simulink model "RBG_Einmassenmodell_Verifikation_Validierung"  (R2021a)
settings: Solver=ode45  StartTime=0.0  StopTime=20  MaxStep=0.02  RelTol=1e-3  EnableMultiTasking=on
settings Model: Creator=beck  LastModifiedBy=Benjamin
settings SolverCC: AlgebraicLoopSolver=TrustRegion
settings DataIOCC: LimitDataPoints=on  SaveFormat=Array  SignalLoggingSaveFormat=ModelDataLogs  ReturnWorkspaceOutputs=off
settings OptimizationCC: ExpressionDepthLimit=2147483647  InitFltsAndDblsToZero=on  LifeSpan=inf
settings DebuggingCC: SaveWithParameterizedLinksMsg=none  UnderspecifiedInitializationDetection=Classic  MergeDetectMultiDrivingBlocksExec=none  SignalResolutionControl=TryResolveAllWithWarning  SolverPrmCheckMsg=warning  FcnCallInpInsideContextMsg=warning  StateNameClashWarn=warning  SFUnexpectedBacktrackingDiag=warning  SFNoUnconditionalDefaultTransitionDiag=warning  SFExecutionAtInitializationDiag=none  SFMachineParentedDataDiag=warning  ArithmeticOperatorsInVariantConditions=warning
settings HardwareCC: ProdBitPerPointer=32  ProdBitPerSizeT=32  ProdBitPerPtrDiffT=32  ProdLargestAtomicFloat=None  ProdIntDivRoundTo=Undefined  ProdEndianess=Unspecified  ProdWordSize=32  ProdHWDeviceType=32-bit Generic
settings ModelReferenceCC: PropagateSignalLabelsOutOfModel=off
settings SFSimCC: SimUseLocalCustomCode=off  CustomCodeUndefinedFunction=UseInterfaceOnly
settings RTWCC: RTWUseLocalCustomCode=off
settings CodeAppCC: StateflowObjectComments=on
settings GRTTargetCC: TargetFcnLib=ansi_tfl_tmw.mat  TargetLangStandard=C89/C90 (ANSI)  CombineOutputUpdateFcns=off  GRTInterface=on
settings ConfigComp: CovMetricSettings=dw  CovSaveCumulativeToWorkspaceVar=on  CovSaveSingleToWorkspaceVar=on  CovExternalEMLEnable=off  CovSFcnEnable=off

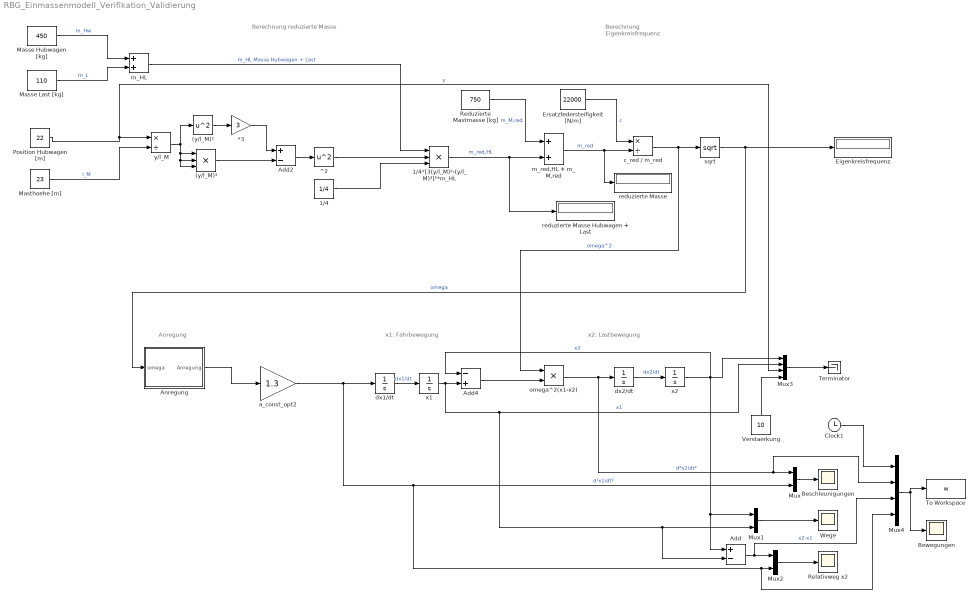
== system RBG_Einmassenmodell_Verifikation_Validierung ==
  note: x2: Lastbewegung
  note: x1: Fahrbewegung
  note: Berechnung
      | reduzierte Masse
  note: Berechnung
      | Eigenkreisfrequenz
  note: Anregung
  (y/l_M)² : Math  Operator=square  SignedPower=on  SaturateOnIntegerOverflow=on
  (y/l_M)³ : Product  Inputs=3  RndMeth=Zero
  *3 : Gain  Gain=3
  1/4 : Constant  Value=1/4
  1/4*[3(y/l_M)²-(y/l_M)³]²*m_HL : Product  Inputs=3  RndMeth=Zero
  Add : Sum  Inputs=+-
  Add2 : Sum  Inputs=+-
  Add4 : Sum  Inputs=-+
  Anregung : Subsystem
  Beschleunigungen : Scope
  Bewegungen : Scope
  Clock1 : Clock
  Eigenkreisfrequenz : Display
  Ersatzfedersteifigkeit [N/m] : Constant  Value=22000
  Masse Hubwagen [kg] : Constant  Value=450
  Masse Last [kg] : Constant  Value=110
  Masthoehe [m] : Constant  Value=23
  Mux : Mux  Inputs=2
  Mux1 : Mux  Inputs=2
  Mux2 : Mux  Inputs=2
  Mux3 : Mux
  Mux4 : Mux
  Position Hubwagen [m] : Constant  Value=22
  Reduzierte Mastmasse [kg] : Constant  Value=750
  Relativweg x2 : Scope
  Terminator : Terminator
  To Workspace : ToWorkspace  VariableName=w  SampleTime=-1
  Verstaerkung : Constant  Value=10
  Wege : Scope
  ^2 : Math  Operator=square  SignedPower=on  SaturateOnIntegerOverflow=on
  a_const_opt2 : Gain  Gain=1.3
  c_red / m_red : Product  Inputs=*/  RndMeth=Zero
  dx1/dt : Integrator
  dx2/dt : Integrator
  m_HL : Sum
  m_red,HL + m_M,red : Sum
  omega^2(x1-x2) : Product  RndMeth=Zero
  reduzierte Masse : Display
      settings: Decimation=2
  reduzierte Masse Hubwagen + Last : Display
      settings: Decimation=2
  sqrt : Math  Operator=sqrt  SignedPower=on  SaturateOnIntegerOverflow=on
  x1 : Integrator
  x2 : Integrator
  y/l_M : Product  Inputs=*/  RndMeth=Zero
  wires:
  Position Hubwagen [m]/1 -> y/l_M/1, Mux3/3  "y"
  Mux/1 -> Beschleunigungen/1
  Mux1/1 -> Wege/1
  Masthoehe [m]/1 -> y/l_M/2  "l_M"
  (y/l_M)²/1 -> *3/1
  *3/1 -> Add2/1
  (y/l_M)³/1 -> Add2/2
  y/l_M/1 -> (y/l_M)³/3, (y/l_M)³/2, (y/l_M)³/1, (y/l_M)²/1
  Ersatzfedersteifigkeit [N/m]/1 -> c_red / m_red/1  "c"
  c_red / m_red/1 -> sqrt/1, omega^2(x1-x2)/1  "omega^2"
  m_red,HL + m_M,red/1 -> reduzierte Masse/1, c_red / m_red/2  "m_red"
  sqrt/1 -> Eigenkreisfrequenz/1, Anregung/1(omega)  "omega"
  omega^2(x1-x2)/1 -> dx2/dt/1, Mux4/2, Mux/1  "d²x2/dt²"
  dx2/dt/1 -> x2/1  "dx2/dt"
  dx1/dt/1 -> x1/1  "dx1/dt"
  Add4/1 -> omega^2(x1-x2)/2
  x1/1 -> Add4/2, Mux1/2, Add/2, Mux3/2  "x1"
  x2/1 -> Add/1, Mux1/1, Mux3/1, Add4/1  "x2"
  Verstaerkung/1 -> Mux3/4
  Add2/1 -> ^2/1
  Reduzierte Mastmasse [kg]/1 -> m_red,HL + m_M,red/1  "m_M,red"
  Mux2/1 -> Relativweg x2/1
  Add/1 -> Mux4/3, Mux2/1  "x2-x1"
  Masse Last [kg]/1 -> m_HL/2  "m_L"
  Masse Hubwagen [kg]/1 -> m_HL/1  "m_Hw"
  1/4*[3(y/l_M)²-(y/l_M)³]²*m_HL/1 -> m_red,HL + m_M,red/2, reduzierte Masse Hubwagen + Last/1  "m_red,HL"
  ^2/1 -> 1/4*[3(y/l_M)²-(y/l_M)³]²*m_HL/2
  m_HL/1 -> 1/4*[3(y/l_M)²-(y/l_M)³]²*m_HL/1  "m_HL Masse Hubwagen + Last"
  1/4/1 -> 1/4*[3(y/l_M)²-(y/l_M)³]²*m_HL/3
  a_const_opt2/1 -> dx1/dt/1, Mux/2, Mux4/4, Mux2/2  "d²x1/dt²"
  Anregung/1(Anregung) -> a_const_opt2/1
  Mux4/1 -> To Workspace/1, Bewegungen/1
  Mux3/1 -> Terminator/1
  Clock1/1 -> Mux4/1

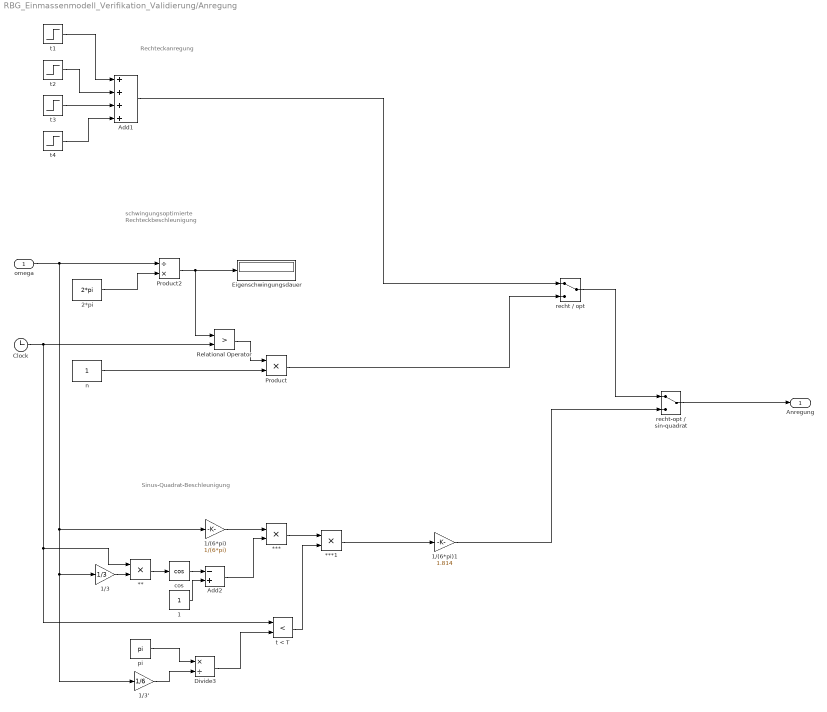
== system RBG_Einmassenmodell_Verifikation_Validierung/Anregung ==
  note: Rechteckanregung
  note: schwingungsoptimierte Rechteckbeschleunigung
  note: Sinus-Quadrat-Beschleunigung
  omega : Inport
  ** : Product  RndMeth=Zero
  *** : Product  RndMeth=Zero
  ***1 : Product  RndMeth=Zero
  1 : Constant
  1/(6*pi) : Gain  Gain=1/(6*pi)
  1/(6*pi)1 : Gain  Gain=1.814
  1/3 : Gain  Gain=1/3
  1/3' : Gain  Gain=1/6
  2*pi : Constant  Value=2*pi
  Add1 : Sum  Inputs=++++
  Add2 : Sum  Inputs=-+
  Clock : Clock
  Divide3 : Product  Inputs=*/
  Eigenschwingungsdauer : Display
  Product : Product  RndMeth=Zero
  Product2 : Product  Inputs=/*  RndMeth=Zero
  Relational Operator : RelationalOperator  Operator=>  RndMeth=Nearest
  "cos " : Trigonometry  Operator=cos
  n : Constant
  pi : Constant  Value=pi
  recht / opt : ManualSwitch
  recht-opt / sin-quadrat : ManualSwitch
  t < T : RelationalOperator  Operator=<  OutDataTypeStr=boolean  RndMeth=Nearest
  t1 : Step  Time=2  SampleTime=0
  t2 : Step  Time=4  After=-1  SampleTime=0
  t3 : Step  Time=15  After=-1  SampleTime=0
  t4 : Step  Time=17  SampleTime=0
  Anregung : Outport
  wires:
  2*pi/1 -> Product2/2
  t1/1 -> Add1/1
  t2/1 -> Add1/2
  Clock/1 -> Relational Operator/2, **/1, t < T/1
  n/1 -> Product/2
  t3/1 -> Add1/3
  t4/1 -> Add1/4
  Product2/1 -> Eigenschwingungsdauer/1, Relational Operator/1
  Relational Operator/1 -> Product/1
  Product/1 -> recht / opt/2
  omega/1 -> Product2/1, 1/(6*pi)/1, 1/3/1, 1/3'/1
  1/3/1 -> **/2
  **/1 -> "cos "/1
  "cos "/1 -> Add2/1
  1/1 -> Add2/2
  1/(6*pi)/1 -> ***/1
  Add2/1 -> ***/2
  ***/1 -> ***1/1
  pi/1 -> Divide3/1
  Divide3/1 -> t < T/2
  t < T/1 -> ***1/2
  recht-opt / sin-quadrat/1 -> Anregung/1
  1/3'/1 -> Divide3/2
  ***1/1 -> 1/(6*pi)1/1
  1/(6*pi)1/1 -> recht-opt / sin-quadrat/2
  Add1/1 -> recht / opt/1
  recht / opt/1 -> recht-opt / sin-quadrat/1
